simulink model "verify_Window_Ventilation_mdl"  (R2018b)
settings: Solver=ode45  StartTime=0.0  StopTime=200  MaxStep=10  RelTol=1e-3  EnableMultiTasking=on
libraries: simulink x1, carnot x1
settings Model: Creator=drhf  LastModifiedBy=drhf
settings DataIOCC: LimitDataPoints=on  SaveFormat=Array  SignalLoggingSaveFormat=ModelDataLogs
settings OptimizationCC: ExpressionDepthLimit=2147483647  LifeSpan=inf
settings DebuggingCC: UnderspecifiedInitializationDetection=Classic  MergeDetectMultiDrivingBlocksExec=none  SolverPrmCheckMsg=warning  FcnCallInpInsideContextMsg=warning  StateNameClashWarn=warning  SFUnexpectedBacktrackingDiag=warning  SFNoUnconditionalDefaultTransitionDiag=warning  SFExecutionAtInitializationDiag=none
settings HardwareCC: ProdBitPerPointer=32  ProdBitPerSizeT=32  ProdBitPerPtrDiffT=32  ProdLargestAtomicFloat=None  ProdIntDivRoundTo=Undefined  ProdEndianess=Unspecified  ProdWordSize=32  ProdHWDeviceType=32-bit Generic
settings ModelReferenceCC: PropagateSignalLabelsOutOfModel=off
settings SFSimCC: SimUseLocalCustomCode=off
settings RTWCC: RTWUseLocalCustomCode=off
settings CodeAppCC: StateflowObjectComments=on
settings GRTTargetCC: TargetLangStandard=C89/C90 (ANSI)  GeneratePreprocessorConditionals=Disable all  CombineOutputUpdateFcns=off  GRTInterface=on
settings ConfigComp: CovMetricSettings=dw  CovHtmlReporting=on  CovSaveCumulativeToWorkspaceVar=on  CovSaveSingleToWorkspaceVar=on  CovExternalEMLEnable=off

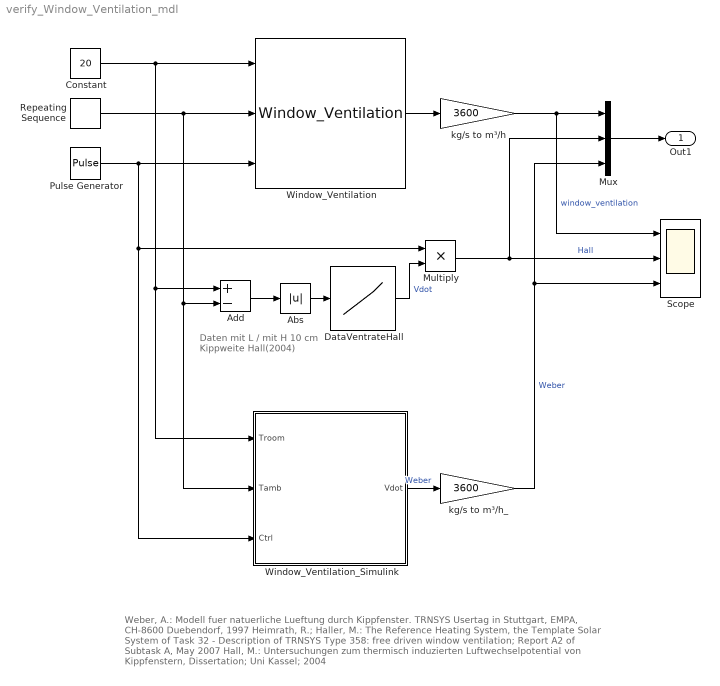
== system verify_Window_Ventilation_mdl ==
  note: Weber, A.: Modell fuer natuerliche Lueftung durch Kippfenster.
      | TRNSYS Usertag in Stuttgart, EMPA, CH-8600 Duebendorf, 1997
      |
      | Heimrath, R.; Haller, M.: The Reference Heating System, the Template Solar System of Task 32
      | - Description of TRNSYS Type 358: free driven window ventilation; Report A2 of Subtask A, May 2007
      |
      | Hall, M.: Untersuchungen zum thermisch induzierten Luftwechselpotential von Kippfenstern,
      | Dissertation; Uni Kassel; 2004
  note: Daten mit L / mit H
      | 10 cm Kippweite
      | Hall(2004)
  Abs : Abs
  Add : Sum  Inputs=+-
  Constant : Constant  Value=20
  DataVentrateHall : Lookup_n-D  NumberOfTableDimensions=1  BreakpointsForDimension1=[0:5:30]  Table=[0 50 65 80 90 100 110]  InternalRulePriority=Speed  RndMeth=Simplest  InputSameDT=on
  Multiply : Product
  Mux : Mux  Inputs=3
  Pulse Generator : DiscretePulseGenerator  PulseType=Time based  Period=200  PulseWidth=50
  Repeating Sequence : simulink/Sources/Repeating Sequence  rep_seq_t=[0 10 90 100]  rep_seq_y=[-10 -10 30 30]
  Scope : Scope  NumInputPorts=3
  Window_Ventilation : carnot/Source/Ventilation/Window_Ventilation  alpha="asin(0.1/1.23)*180/pi  % 10 cm Kippweite"  H=1.23  W=0.94  Nwin=1
      settings: SourceProductName=Carnot
  Window_Ventilation_Simulink : Subsystem  mask(window ventilation){Alpha=asin(0.1/1.23)*180/pi  % 10 cm Kippweite, H=1.23, W=0.93, Nwin=1}
      mask prompts: Alpha "Maximal opening angle  in °"; H "Height of window in m"; W "Width of window in m"; Nwin "Number of windows"
      mask help: Simulates the free driven ventilation through a window with an opening angle of [0,1]* max. angle. Valid for angles between 8° and 180°. Output is the VOLUME FLOW RATE in m^3/s. Calculation based on Weber.
      mask Help: web(fullfile(path_carnot('help'),'Window_Ventilation.html'),'-helpbrowser')
      mask TypeOptions Alpha: Alpha/Gain
      mask TypeOptions H: Height1/Value | Height2/Gain | Height3/Value
      mask TypeOptions W: Width1/Gain | Width2/Value
      mask TypeOptions Nwin: NumberOfWindows/Gain
      mask Display:
      | plot(0,10,90,80,[20 70 70 20 20],[20 20 70 70 20],...
      |     [20 70 80 30 20],[20 20 65 65 20])
  kg/s to m³/h : Gain  Gain=3600
  kg/s to m³/h_ : Gain  Gain=3600
  Out1 : Outport
  wires:
  Window_Ventilation/1 -> kg/s to m³/h/1
  Constant/1 -> Window_Ventilation/1, Window_Ventilation_Simulink/1(Troom), Add/1
  Pulse Generator/1 -> Window_Ventilation/3, Window_Ventilation_Simulink/3(Ctrl), Multiply/1
  Repeating Sequence/1 -> Window_Ventilation/2, Window_Ventilation_Simulink/2(Tamb), Add/2
  Add/1 -> Abs/1
  Abs/1 -> DataVentrateHall/1
  Mux/1 -> Out1/1
  Multiply/1 -> Mux/2, Scope/2  "Hall"
  Window_Ventilation_Simulink/1(Vdot) -> kg/s to m³/h_/1  "Weber"
  DataVentrateHall/1 -> Multiply/2  "Vdot"
  kg/s to m³/h/1 -> Scope/1, Mux/1  "window_ventilation"
  kg/s to m³/h_/1 -> Mux/3, Scope/3  "Weber"

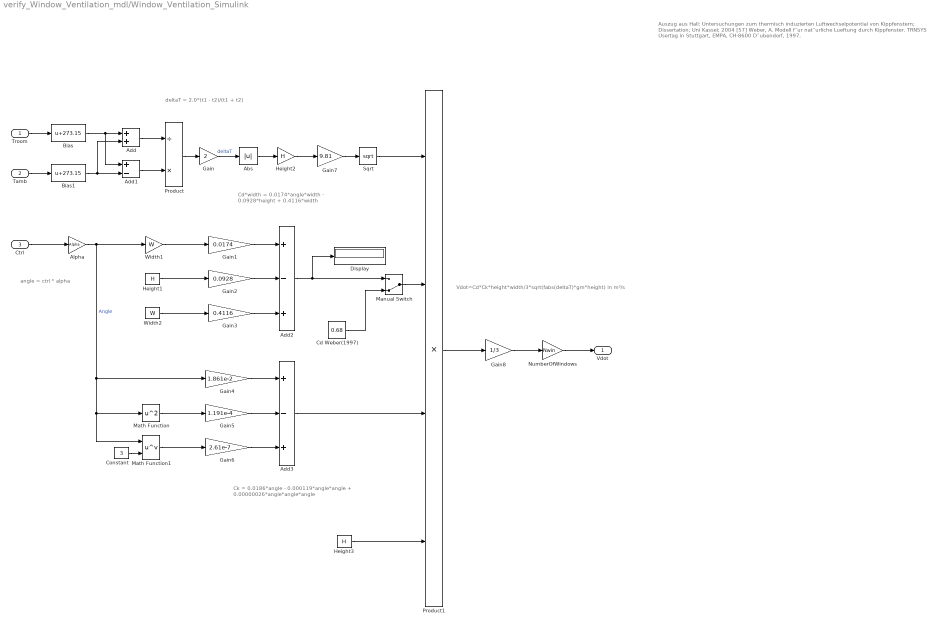
== system verify_Window_Ventilation_mdl/Window_Ventilation_Simulink ==
  note: Vdot=Cd*Ck*height*width/3*sqrt(fabs(deltaT)*gm*height)
      | in m³/s
  note: angle = ctrl * alpha
  note: Ck = 0.0186*angle
      | - 0.000119*angle*angle
      | + 0.00000026*angle*angle*angle
  note: Auszug aus
      | Hall: Untersuchungen zum thermisch induzierten Luftwechselpotential von Kippfenstern; Dissertation;
      | Uni Kassel; 2004
      | [57] Weber, A. Modell f¨ur nat¨urliche Lueftung durch Kippfenster. TRNSYS Usertag
      | in Stuttgart, EMPA, CH-8600 D¨ubendorf, 1997.
  note: Cd*width = 0.0174*angle*width
      | - 0.0928*height + 0.4116*width
  note: deltaT = 2.0*(t1 - t2)/(t1 + t2)
  Troom : Inport
  Tamb : Inport  Port=2
  Ctrl : Inport  Port=3
  Abs : Abs
  Add : Sum
  Add1 : Sum  Inputs=+-
  Add2 : Sum  Inputs=+-+
  Add3 : Sum  Inputs=+-+
  Alpha : Gain  Gain=Alpha
  Bias : Bias  Bias=273.15
  Bias1 : Bias  Bias=273.15
  Cd Weber(1997) : Constant  Value=0.68
  Constant : Constant  Value=3
  Display : Display
  Gain : Gain  Gain=2
  Gain1 : Gain  Gain=0.0174
  Gain2 : Gain  Gain=0.0928
  Gain3 : Gain  Gain=0.4116
  Gain4 : Gain  Gain=1.861e-2
  Gain5 : Gain  Gain=1.191e-4
  Gain6 : Gain  Gain=2.61e-7
  Gain7 : Gain  Gain=9.81
  Gain8 : Gain  Gain=1/3
  Height1 : Constant  Value=H
  Height2 : Gain  Gain=H
  Height3 : Constant  Value=H
  Manual Switch : ManualSwitch  CurrentSetting=0
  Math Function : Math  Operator=square  SaturateOnIntegerOverflow=on
  Math Function1 : Math  Operator=pow  SaturateOnIntegerOverflow=on
  NumberOfWindows : Gain  Gain=Nwin
  Product : Product  Inputs=/*
  Product1 : Product  Inputs=4
  Sqrt : Sqrt  SaturateOnIntegerOverflow=on
  Width1 : Gain  Gain=W
  Width2 : Constant  Value=W
  Vdot : Outport
  wires:
  NumberOfWindows/1 -> Vdot/1
  Ctrl/1 -> Alpha/1
  Alpha/1 -> Width1/1, Math Function1/1, Math Function/1, Gain4/1  "Angle"
  Troom/1 -> Bias/1
  Tamb/1 -> Bias1/1
  Add/1 -> Product/1
  Add1/1 -> Product/2
  Product/1 -> Gain/1
  Gain/1 -> Abs/1  "deltaT"
  Width1/1 -> Gain1/1
  Height1/1 -> Gain2/1
  Gain2/1 -> Add2/2
  Gain3/1 -> Add2/3
  Width2/1 -> Gain3/1
  Gain4/1 -> Add3/1
  Math Function/1 -> Gain5/1
  Constant/1 -> Math Function1/2
  Gain5/1 -> Add3/2
  Math Function1/1 -> Gain6/1
  Gain6/1 -> Add3/3
  Abs/1 -> Height2/1
  Height2/1 -> Gain7/1
  Gain7/1 -> Sqrt/1
  Product1/1 -> Gain8/1
  Gain8/1 -> NumberOfWindows/1
  Sqrt/1 -> Product1/1
  Add2/1 -> Display/1, Manual Switch/1
  Height3/1 -> Product1/4
  Gain1/1 -> Add2/1
  Add3/1 -> Product1/3
  Bias/1 -> Add1/1, Add/1
  Bias1/1 -> Add/2, Add1/2
  Cd Weber(1997)/1 -> Manual Switch/2
  Manual Switch/1 -> Product1/2
